simulink model "TransferFunc"  (R2015a)
settings: Solver=ode4  StartTime=0.0  StopTime=100  FixedStep=0.002  RelTol=1e-3
undefined symbols (not defined in the file or in its folder): ans
settings Model: Creator=Andrew  LastModifiedBy=12cfh
settings DebuggingCC: UnderspecifiedInitializationDetection=Classic  MergeDetectMultiDrivingBlocksExec=none  SolverPrmCheckMsg=warning  StateNameClashWarn=warning

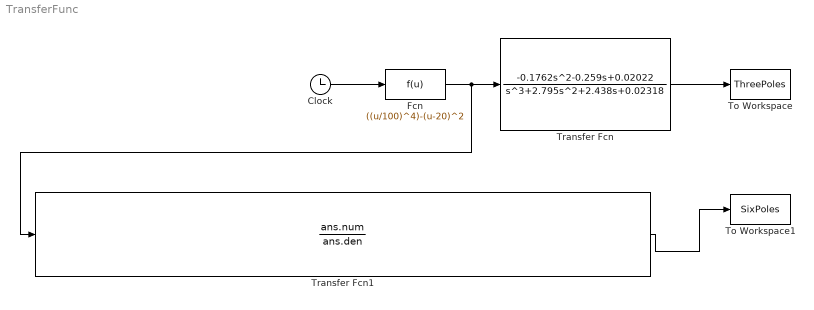
== system TransferFunc ==
  Clock : Clock
  Fcn : Fcn  Expr=((u/100)^4)-(u-20)^2
  To Workspace : ToWorkspace  VariableName=ThreePoles  SaveFormat=Structure With Time  SampleTime=-1
  To Workspace1 : ToWorkspace  VariableName=SixPoles  SaveFormat=Structure With Time  SampleTime=-1
  Transfer Fcn : TransferFcn  Numerator=[0 -0.1762 -0.259 0.02022]  Denominator=[1 2.795 2.438 0.02318]
  Transfer Fcn1 : TransferFcn  Numerator=ans.num  Denominator=ans.den
  wires:
  Clock/1 -> Fcn/1
  Fcn/1 -> Transfer Fcn1/1, Transfer Fcn/1
  Transfer Fcn/1 -> To Workspace/1
  Transfer Fcn1/1 -> To Workspace1/1
